simulink model "uidread_host_demo"  (Simulink 7.3)
settings: Solver=FixedStepDiscrete  SolverMode=SingleTasking  StartTime=0.0  StopTime=10.0  RelTol=1e-3
PreLoadFcn:
  | waijung.modelPreload; % Required for working with Waijung Blockset. Do not remove.
CloseFcn:
  | waijung.modelClose; % Required for working with Waijung Blockset. Do not remove.
settings Model: Creator=Krisada  LastModifiedBy=Krisada
settings OptimizationCC: OptimizeModelRefInitCode=on  LifeSpan=1
settings HardwareCC: ProdEndianess=LittleEndian  ProdHWDeviceType=ARM Compatible->Cortex - M4  TargetEndianess=LittleEndian  TargetHWDeviceType=ARM Compatible->Cortex - M4
settings RTWCC: SystemTargetFile=stm32f4.tlc  GenerateMakefile=off  TemplateMakefile=ert_default_tmf  Description=STM32F4 Target  ProcessScript=stm32f4_make_rtw_hook
settings CodeAppCC: IgnoreCustomStorageClasses=off
settings STFCustomTargetCC: ModelReferenceCompliant=off  CombineOutputUpdateFcns=on  ERTCustomFileBanners=on  SupportContinuousTime=off  SupportNonInlinedSFcns=off  SystemTargetFile=stm32f4.tlc
settings ERTTargetCC: MultiwordLength=2048  ModelReferenceCompliant=off  ParMdlRefBuildCompliant=off  CompOptLevelCompliant=off  ERTFirstTimeCompliant=off  ModelStepFunctionPrototypeControlCompliant=off  CPPClassGenCompliant=off  ExtModeMexFile=noextcomm  InlinedParameterPlacement=NonHierarchical  ERTSrcFileBannerTemplate=stm32f4_code_template.cgt  ERTHdrFileBannerTemplate=stm32f4_code_template.cgt  ERTDataSrcFileTemplate=stm32f4_code_template.cgt  ERTDataHdrFileTemplate=stm32f4_code_template.cgt  ERTCustomFileTemplate=stm32f4_file_process.tlc

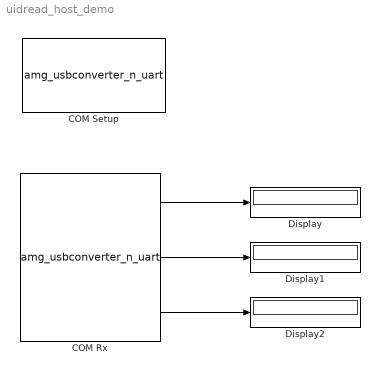
== system uidread_host_demo ==
  COM Rx : S-Function  FunctionName=amg_usbconverter_n_uart  Parameters=id,port,setup_baudrate,setup_databits,setup_parity,setup_stopbits,setup_timeout,packetmode,ascii_printf_format,ascii_typecastarray,ascii_typecastcount,bin_headerarray,bin_headercount,bin_terminatorarray,bin_terminatorcount,bin_datatypearray,bin_datatypecount,sampletime,sampletimestr,blockid  EnableBusSupport=off  mask(amg_usbconverter_n_uart){id=rx, port=COM10, setup_baudrate=115200, setup_databits=8, setup_parity=Odd, setup_stopbits=1, setup_timeout=10000, packetmode=Binary, bin_header='7E 7E', bin_datalength=12, d1datatype=uint32, d2datatype=uint32, d3datatype=uint32, d4datatype=not used, d5datatype=not used, d6datatype=not used, d7datatype=not used, d8datatype=not used, d9datatype=not used, d10datatype=not used, d11datatype=not used, d12datatype=not used, d13datatype=not used, d14datatype=not used, d15datatype=not used, d16datatype=not used, bin_terminator='03 03', ascii_format='Value=%d', ascii_endofpacket=LF (0x0A - "\n"), ascii_printf_format=Value=%d, ascii_typecastarray=[ "","int32_t"], ascii_typecastcount=1, bin_headerarray=[126  126], bin_headercount=2, bin_terminatorarray=[3  3], bin_terminatorcount=2, bin_datatypearray=[7  7  7  1  0  0  0  1  0  0  0  1  0  0  0  0], bin_datatypecount=3, sampletime=0.02, sampletimestr=0.02, blockid=uidread_host_demoCOMRx}
      mask prompts: setup_baudrate "Baud Rate"; setup_databits "Data Bits"; setup_parity "Parity"; setup_stopbits "Stop Bits"; setup_timeout "Timeout (mS)"; packetmode "Packet mode"; bin_header "Header (example: '7E 7E')"; bin_datalength "Data length (bytes)"; d1datatype "D1 Data Type"; d2datatype "D2 Data Type"; d3datatype "D3 Data Type"; d4datatype "D4 Data Type"; d5datatype "D5 Data Type"; d6datatype "D6 Data Type"; d7datatype "D7 Data Type"; d8datatype "D8 Data Type"; d9datatype "D9 Data Type"; d10datatype "D10 Data Type"; d11datatype "D11 Data Type"; d12datatype "D12 Data Type"; d13datatype "D13 Data Type"; d14datatype "D14 Data Type"; d15datatype "D15 Data Type"; d16datatype "D16 Data Type"; bin_terminator "Terminator (example: '03 03')"; ascii_format "Format"; ascii_endofpacket "End of packet"; ascii_printf_format "Ascii print format"; ascii_typecastarray "Ascii type cast array"; ascii_typecastcount "Ascii type cast count"; bin_headerarray "Header array"; bin_headercount "Header count"; bin_terminatorarray "Terminator array"; bin_terminatorcount "Terminator count"; bin_datatypearray "Data type array"; bin_datatypecount "Data type count"; sampletime "Sample time (sec)"; sampletimestr "Compiled sample time (sec) in string"
      mask init:
      | amg_usbconverter_n_uart_callback('init');
      mask Help: web(fullfile(waijungdocroot,'amg_usbconverter_n_uart.htm'), '-browser')
      mask StyleString: popup(setup|tx|rx),popup(COM3|COM10|COM11),edit,edit,popup(None|Odd|Even),popup(1|1.5|2),edit,popup(Binary|Ascii),edit,edit,popup(double|single|uint32|int32|uint16|int16|uint8|int8),popup(not used|double|single|uint32|int32|uint16|int16|uint8|int8),popup(not used|double|single|uint32|int32|uint16|int16|uint8|int8),popup(not used|double|single|uint32|int32|uint16|int16|uint8|int8),popup(not used|double|single|uint32|int32|uint16|int16|uint8|int8),popup(not used|double|single|uint32|int32|uint16|int16|uint8|int8),popup(not used|double|single|uint32|int32|uint16|int16|uint8|int8),popup(not used|double|single|uint32|int32|uint16|int16|uint8|int8),popup(not used|double|single|uint32|int32|uint16|int16|uint8|int8),popup(not used|double|single|uint32|int32|uint16|int16|uint8|int8),popup(not used|double|single|uint32|int32|uint16|int16|uint8|int8),popup(not used|double|single|uint32|int32|uint16|int16|uint8|int8),popup(not used|double|single|uint32|int32|uint16|int16|uint8|int8),popup(not used|double|single|uint32|int32|uint16|int16|uint8|int8),popup(not used|double|single|uint32|int32|uint16|int16|uint8|int8),popup(not used|double|single|uint32|int32|uint16|int16|uint8|int8),edit,edit,popup(CR (0x0D - "\r")|LF (0x0A - "\n")|CRLF (0x0D 0x0A - "\r\n")|None),edit,edit,edit,edit,edit,edit,edit,edit,edit,edit,edit,edit
      mask CallbackString: amg_usbconverter_n_uart_callback('id');|amg_usbconverter_n_uart_callback('port');||||||amg_usbconverter_n_uart_callback('packetmode');|amg_usbconverter_n_uart_callback('bin_header');||amg_usbconverter_n_uart_callback('d1datatype');|amg_usbconverter_n_uart_callback('d2datatype');|amg_usbconverter_n_uart_callback('d3datatype');|amg_usbconverter_n_uart_callback('d4datatype');|amg_usbconverter_n_uart_callback('d5datatype');|amg_usbconverter_n_uart_callback('d6datatype');|amg_usbconverter_n_uart_callback('d7datatype');|amg_usbconverter_n_uart_callback('d8datatype');|amg_usbconverter_n_uart_callback('d9datatype');|amg_usbconverter_n_uart_callback('d10datatype');|amg_usbconverter_n_uart_callback('d11datatype');|amg_usbconverter_n_uart_callback('d12datatype');|amg_usbconverter_n_uart_callback('d13datatype');|amg_usbconverter_n_uart_callback('d14datatype');|amg_usbconverter_n_uart_callback('d15datatype');|amg_usbconverter_n_uart_callback('d16datatype');|amg_usbconverter_n_uart_callback('bin_terminator');|amg_usbconverter_n_uart_callback('ascii_format');|||||||||||amg_usbconverter_n_uart_callback('sampletime');|amg_usbconverter_n_uart_callback('sampletimestr');|amg_usbconverter_n_uart_callback('blockid');
      mask Display: text(0.05, 0.5, '[COM10]\nPacket: Binary\nTs (sec): 0.02','ver','middle','hor','left')port_label('output', 1,'uint32')port_label('output', 2,'uint32')port_label('output', 3,'uint32')
  COM Setup : S-Function  FunctionName=amg_usbconverter_n_uart  Parameters=id,port,setup_baudrate,setup_databits,setup_parity,setup_stopbits,setup_timeout,packetmode,ascii_printf_format,ascii_typecastarray,ascii_typecastcount,bin_headerarray,bin_headercount,bin_terminatorarray,bin_terminatorcount,bin_datatypearray,bin_datatypecount,sampletime,sampletimestr,blockid  EnableBusSupport=off  mask(amg_usbconverter_n_uart){id=setup, port=COM10, setup_baudrate=115200, setup_databits=8, setup_parity=None, setup_stopbits=1, setup_timeout=1000, packetmode=Binary, bin_header='7E 7E', bin_datalength=12, d1datatype=uint32, d2datatype=double, d3datatype=not used, d4datatype=not used, d5datatype=not used, d6datatype=not used, d7datatype=not used, d8datatype=not used, d9datatype=not used, d10datatype=not used, d11datatype=not used, d12datatype=not used, d13datatype=not used, d14datatype=not used, d15datatype=not used, d16datatype=not used, bin_terminator='03 03', ascii_format='Value=%d', ascii_endofpacket=LF (0x0A - "\n"), ascii_printf_format=Value=%d, ascii_typecastarray=[ "","int32_t"], ascii_typecastcount=1, bin_headerarray=[126  126], bin_headercount=2, bin_terminatorarray=[3  3], bin_terminatorcount=2, bin_datatypearray=[7  0  1  1  0  0  0  1  0  0  0  1  0  0  0  0], bin_datatypecount=2, sampletime=inf, sampletimestr=0.02, blockid=uidread_host_demoCOMSetup}
      mask prompts: setup_baudrate "Baud Rate"; setup_databits "Data Bits"; setup_parity "Parity"; setup_stopbits "Stop Bits"; setup_timeout "Timeout (mS)"; packetmode "Packet mode"; bin_header "Header (example: '7E 7E')"; bin_datalength "Data length (bytes)"; d1datatype "D1 Data Type"; d2datatype "D2 Data Type"; d3datatype "D3 Data Type"; d4datatype "D4 Data Type"; d5datatype "D5 Data Type"; d6datatype "D6 Data Type"; d7datatype "D7 Data Type"; d8datatype "D8 Data Type"; d9datatype "D9 Data Type"; d10datatype "D10 Data Type"; d11datatype "D11 Data Type"; d12datatype "D12 Data Type"; d13datatype "D13 Data Type"; d14datatype "D14 Data Type"; d15datatype "D15 Data Type"; d16datatype "D16 Data Type"; bin_terminator "Terminator (example: '03 03')"; ascii_format "Format"; ascii_endofpacket "End of packet"; ascii_printf_format "Ascii print format"; ascii_typecastarray "Ascii type cast array"; ascii_typecastcount "Ascii type cast count"; bin_headerarray "Header array"; bin_headercount "Header count"; bin_terminatorarray "Terminator array"; bin_terminatorcount "Terminator count"; bin_datatypearray "Data type array"; bin_datatypecount "Data type count"; sampletime "Sample time (sec)"; sampletimestr "Compiled sample time (sec) in string"
      mask init:
      | amg_usbconverter_n_uart_callback('init');
      mask Help: web(fullfile(waijungdocroot,'amg_usbconverter_n_uart.htm'), '-browser')
      mask StyleString: popup(setup|tx|rx),popup(COM3|COM10|COM11),edit,edit,popup(None|Odd|Even),popup(1|1.5|2),edit,popup(Binary|Ascii),edit,edit,popup(double|single|uint32|int32|uint16|int16|uint8|int8),popup(not used|double|single|uint32|int32|uint16|int16|uint8|int8),popup(not used|double|single|uint32|int32|uint16|int16|uint8|int8),popup(not used|double|single|uint32|int32|uint16|int16|uint8|int8),popup(not used|double|single|uint32|int32|uint16|int16|uint8|int8),popup(not used|double|single|uint32|int32|uint16|int16|uint8|int8),popup(not used|double|single|uint32|int32|uint16|int16|uint8|int8),popup(not used|double|single|uint32|int32|uint16|int16|uint8|int8),popup(not used|double|single|uint32|int32|uint16|int16|uint8|int8),popup(not used|double|single|uint32|int32|uint16|int16|uint8|int8),popup(not used|double|single|uint32|int32|uint16|int16|uint8|int8),popup(not used|double|single|uint32|int32|uint16|int16|uint8|int8),popup(not used|double|single|uint32|int32|uint16|int16|uint8|int8),popup(not used|double|single|uint32|int32|uint16|int16|uint8|int8),popup(not used|double|single|uint32|int32|uint16|int16|uint8|int8),popup(not used|double|single|uint32|int32|uint16|int16|uint8|int8),edit,edit,popup(CR (0x0D - "\r")|LF (0x0A - "\n")|CRLF (0x0D 0x0A - "\r\n")|None),edit,edit,edit,edit,edit,edit,edit,edit,edit,edit,edit,edit
      mask CallbackString: amg_usbconverter_n_uart_callback('id');|amg_usbconverter_n_uart_callback('port');||||||amg_usbconverter_n_uart_callback('packetmode');|amg_usbconverter_n_uart_callback('bin_header');||amg_usbconverter_n_uart_callback('d1datatype');|amg_usbconverter_n_uart_callback('d2datatype');|amg_usbconverter_n_uart_callback('d3datatype');|amg_usbconverter_n_uart_callback('d4datatype');|amg_usbconverter_n_uart_callback('d5datatype');|amg_usbconverter_n_uart_callback('d6datatype');|amg_usbconverter_n_uart_callback('d7datatype');|amg_usbconverter_n_uart_callback('d8datatype');|amg_usbconverter_n_uart_callback('d9datatype');|amg_usbconverter_n_uart_callback('d10datatype');|amg_usbconverter_n_uart_callback('d11datatype');|amg_usbconverter_n_uart_callback('d12datatype');|amg_usbconverter_n_uart_callback('d13datatype');|amg_usbconverter_n_uart_callback('d14datatype');|amg_usbconverter_n_uart_callback('d15datatype');|amg_usbconverter_n_uart_callback('d16datatype');|amg_usbconverter_n_uart_callback('bin_terminator');|amg_usbconverter_n_uart_callback('ascii_format');|||||||||||amg_usbconverter_n_uart_callback('sampletime');|amg_usbconverter_n_uart_callback('sampletimestr');|amg_usbconverter_n_uart_callback('blockid');
      mask Display: text(0.5, 0.5, '[COM10]\nBaud: 115200\nFrame: 8-None-1\nTs (sec): 0.02','ver','middle','hor','center')
  Display : Display
      settings: Format=hex (Stored Integer)
  Display1 : Display
      settings: Format=hex (Stored Integer)
  Display2 : Display
      settings: Format=hex (Stored Integer)
  wires:
  COM Rx/1 -> Display/1
  COM Rx/2 -> Display1/1
  COM Rx/3 -> Display2/1
